simulink model "writeJoints"  (Simulink 8.7)
settings: Solver=ode45  StartTime=0.0  StopTime=10.0  RelTol=1e-3
libraries: WBCLibrary x2
settings Model: Creator=luca  LastModifiedBy=gnava
settings DebuggingCC: UnderspecifiedInitializationDetection=Simplified  MergeDetectMultiDrivingBlocksExec=error  SolverPrmCheckMsg=warning
settings ConfigComp: CovSFcnEnable=off

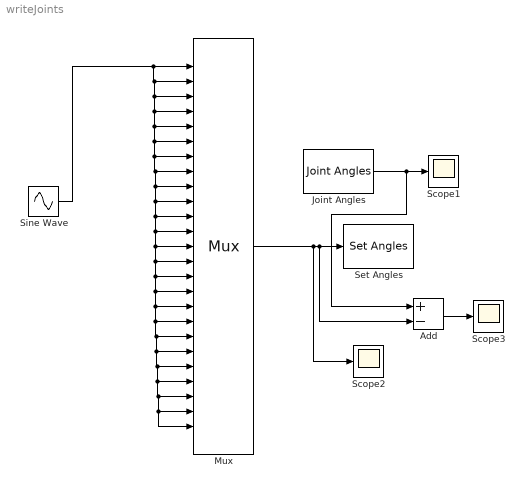
== system writeJoints ==
  Add : Sum  Inputs=+-
  Joint Angles : WBCLibrary/wholeBodyStates/Joint Angles  robotName=robotName  localName=localName
  Mux : Mux  Inputs=25
  Scope1 : Scope
  Scope2 : Scope
  Scope3 : Scope
  Set Angles : WBCLibrary/wholeBodyActuators/Set Angles  val=5  robotName=robotName  localName=localName
  Sine Wave : Sin  SampleTime=0
  wires:
  Sine Wave/1 -> Mux/1, Mux/3, Mux/8, Mux/10, Mux/12, Mux/17, Mux/19, Mux/20, Mux/25, Mux/24, Mux/23, Mux/22, Mux/21, Mux/18, Mux/16, Mux/15, Mux/14, Mux/13, Mux/11, Mux/9, Mux/7, Mux/6, Mux/5, Mux/4, Mux/2
  Joint Angles/1 -> Add/1, Scope1/1
  Mux/1 -> Scope2/1, Add/2, Set Angles/1
  Add/1 -> Scope3/1
